simulink model "FeedbackControl_observer_descrete"  (R2018b)
settings: Solver=VariableStepAuto  StartTime=0.0  StopTime=3.0  RelTol=1e-3
values from neighbouring files (symbols this model uses):
  K = lqr(sys_A, sys_B, Q, R)    [LQRadjuster.m]
  x0 = [20*pi/180;0;0;0]    [LQRadjuster.m]
undefined symbols (not defined in the file or in its folder): sys_Ad, sys_Bd, sys_C, sys_D, Ts
settings Model: Creator=ku_sk  LastModifiedBy=ku_sk

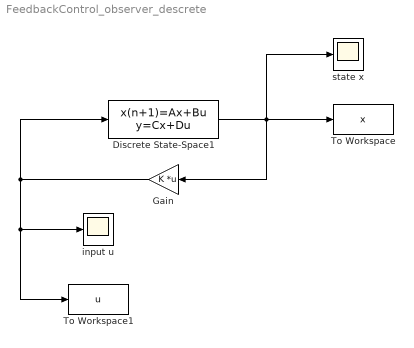
== system FeedbackControl_observer_descrete ==
  Discrete State-Space1 : DiscreteStateSpace  A=sys_Ad  B=sys_Bd  C=sys_C  D=sys_D  InitialCondition=x0  SampleTime=Ts
  Gain : Gain  Gain=K  Multiplication=Matrix(K*u)
  To Workspace : ToWorkspace  VariableName=x  SampleTime=-1
  To Workspace1 : ToWorkspace  VariableName=u  SampleTime=-1
  input u : Scope
  state x : Scope
  wires:
  Discrete State-Space1/1 -> To Workspace/1, state x/1, Gain/1
  Gain/1 -> To Workspace1/1, input u/1, Discrete State-Space1/1
